simulink model "acrobot_sim_v3"  (R2013a)
settings: Solver=ode1  StartTime=0.0  StopTime=10.0  FixedStep=0.1  RelTol=1e-3
PreLoadFcn:
  | m1 = 1;
  | m2 = 1;
  | l1 = 1;
  | l2 = 1;
  | lc1 = l1/2;
  | lc2 = l2/2;
  | Ic1 = (lc1*lc1)/3;
  | Ic2 = (lc2*lc2)/3;
  | I1 = Ic1+m1*lc1*lc1;
  | I2 = Ic2+m2*lc2*lc2;
  | b1 = 0.4;
  | b2 = 0.4;
  | g = 9.8;
StartFcn:
  | m1 = 1;
  | m2 = 1;
  | l1 = 1;
  | l2 = 1;
  | lc1 = l1/2;
  | lc2 = l2/2;
  | Ic1 = (lc1*lc1)/3;
  | Ic2 = (lc2*lc2)/3;
  | I1 = Ic1+m1*lc1*lc1;
  | I2 = Ic2+m2*lc2*lc2;
  | b1 = 0.4;
  | b2 = 0.4;
  | g = 9.8;
libraries: mblibv1 x8, simulink x2
settings Model: Creator=nightling  LastModifiedBy=nightling
settings SimMechanicsCC: VisDuringSimulation=on

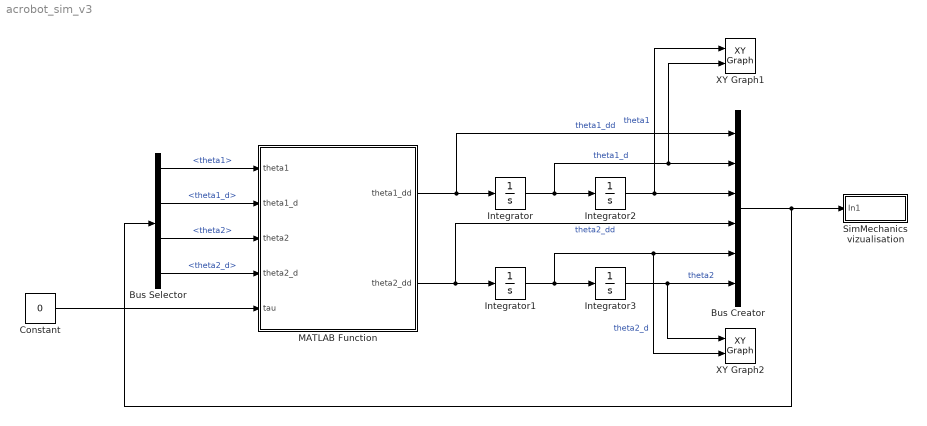
== system acrobot_sim_v3 ==
  Bus Creator : BusCreator  Inputs=6
  Bus Selector : BusSelector  OutputSignals=theta1,theta1_d,theta2,theta2_d
  Constant : Constant  Value=0
  Integrator : Integrator  InitialCondition=[0 ]
  Integrator1 : Integrator  InitialCondition=[0 ]
  Integrator2 : Integrator  InitialCondition=pi/2
  Integrator3 : Integrator  InitialCondition=[0 ]
  MATLAB Function : MATLAB Function  TreatAsAtomicUnit=on
  SimMechanics vizualisation : Subsystem
  XY Graph1 : simulink/Sinks/XY Graph  xmin=-1  xmax=1  ymin=-5  ymax=5  st=-1
  XY Graph2 : simulink/Sinks/XY Graph  xmin=-1  xmax=1  ymin=-5  ymax=5  st=-1
  wires:
  MATLAB Function/1(theta1_dd) -> Bus Creator/1, Integrator/1  "theta1_dd"
  MATLAB Function/2(theta2_dd) -> Integrator1/1, Bus Creator/4  "theta2_dd"
  Integrator/1 -> XY Graph1/2, Bus Creator/2, Integrator2/1  "theta1_d"
  Integrator1/1 -> Integrator3/1, XY Graph2/2, Bus Creator/5  "theta2_d"
  Integrator2/1 -> Bus Creator/3, XY Graph1/1  "theta1"
  Integrator3/1 -> XY Graph2/1, Bus Creator/6  "theta2"
  Constant/1 -> MATLAB Function/5(tau)
  Bus Creator/1 -> Bus Selector/1, SimMechanics vizualisation/1(In1)
  Bus Selector/1 -> MATLAB Function/1(theta1)  "<theta1>"
  Bus Selector/3 -> MATLAB Function/3(theta2)  "<theta2>"
  Bus Selector/2 -> MATLAB Function/2(theta1_d)  "<theta1_d>"
  Bus Selector/4 -> MATLAB Function/4(theta2_d)  "<theta2_d>"

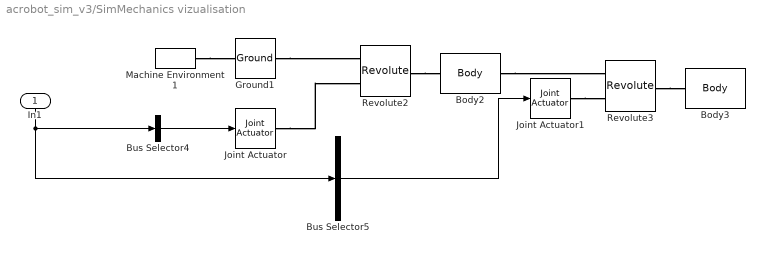
== system acrobot_sim_v3/SimMechanics vizualisation ==
  In1 : Inport
  Body2 : mblibv1/Bodies/Body  LConnTagsString=CS1  RConnTagsString=CS2  UpdateFromCAD=off  DialogClass=MechanicalBodyBlock  Mass=m1  MassUnits=kg  InertiaUnits=kg*m^2  Inertia=zeros(3)  Shape=Cylinder  ShapeDims=[1 1]  ShapeUnits=m  ShapeUse=false  Density=1  DensityUnits=kg/m^3  DensityUse=false  GraphicsMode=MACHINE_DEFAULT  BodyColorSelMode=COLORPALETTE  BodyColor=[0.043137 0.51765 0.78039]  AttachedToCS=CG  CG=Left$CG$[0 -l1/2 0]$CS1$CS1$m$[0 0 0]$Euler X-Y-Z$deg$WORLD$false$none  WorkingFrames=Left$CS1$[0 0 0]$Adjoining$Adjoining$m$[0 0 0]$Euler X-Y-Z$deg$WORLD$true$none#Right$CS2$[0 -l1 0]$CS1$CS1$m$[0 0 0]$Euler X-Y-Z$deg$WORLD$true$none  CGPos=[0 -l1/2 0]  CGRot=[0 0 0]  CS0Pos=[]  CS0Rot=[]  CS1Pos=[0 0 0]  CS1Rot=[0 0 0]  CS2Pos=[0 -l1 0]  CS2Rot=[0 0 0]  CS3Pos=[]  CS3Rot=[]  CS4Pos=[]  CS4Rot=[]  CS5Pos=[]  CS5Rot=[]  CS6Pos=[]  CS6Rot=[]  CS7Pos=[]  CS7Rot=[]  CS8Pos=[]  CS8Rot=[]  CS9Pos=[]  CS9Rot=[]  CS10Pos=[]  CS10Rot=[]  CS11Pos=[]  CS11Rot=[]  CS12Pos=[]  CS12Rot=[]  CS13Pos=[]  CS13Rot=[]  CS14Pos=[]  CS14Rot=[]  CS15Pos=[]  CS15Rot=[]  CS16Pos=[]  CS16Rot=[]  CS17Pos=[]  CS17Rot=[]  CS18Pos=[]  CS18Rot=[]  CS19Pos=[]  CS19Rot=[]  CS20Pos=[]  CS20Rot=[]
  Body3 : mblibv1/Bodies/Body  LConnTagsString=CS1  UpdateFromCAD=off  DialogClass=MechanicalBodyBlock  Mass=m2  MassUnits=kg  InertiaUnits=kg*m^2  Inertia=zeros(3)  Shape=Cylinder  ShapeDims=[1 1]  ShapeUnits=m  ShapeUse=false  Density=1  DensityUnits=kg/m^3  DensityUse=false  GraphicsMode=MACHINE_DEFAULT  BodyColorSelMode=COLORPALETTE  BodyColor=[0.043137 0.51765 0.78039]  AttachedToCS=CG  CG=Left$CG$[0 -l2/2 0]$CS1$CS1$m$[0 0 0]$Euler X-Y-Z$deg$WORLD$false$none  WorkingFrames=Left$CS1$[0 0 0]$Adjoining$Adjoining$m$[0 0 0]$Euler X-Y-Z$deg$WORLD$true$none#Right$CS2$[0 -l2 0]$CS1$CS1$m$[0 0 0]$Euler X-Y-Z$deg$WORLD$false$none  CGPos=[0 -l2/2 0]  CGRot=[0 0 0]  CS0Pos=[]  CS0Rot=[]  CS1Pos=[0 0 0]  CS1Rot=[0 0 0]  CS2Pos=[0 -l2 0]  CS2Rot=[0 0 0]  CS3Pos=[]  CS3Rot=[]  CS4Pos=[]  CS4Rot=[]  CS5Pos=[]  CS5Rot=[]  CS6Pos=[]  CS6Rot=[]  CS7Pos=[]  CS7Rot=[]  CS8Pos=[]  CS8Rot=[]  CS9Pos=[]  CS9Rot=[]  CS10Pos=[]  CS10Rot=[]  CS11Pos=[]  CS11Rot=[]  CS12Pos=[]  CS12Rot=[]  CS13Pos=[]  CS13Rot=[]  CS14Pos=[]  CS14Rot=[]  CS15Pos=[]  CS15Rot=[]  CS16Pos=[]  CS16Rot=[]  CS17Pos=[]  CS17Rot=[]  CS18Pos=[]  CS18Rot=[]  CS19Pos=[]  CS19Rot=[]  CS20Pos=[]  CS20Rot=[]
  Bus Selector4 : BusSelector  OutputSignals=theta1,theta1_d,theta1_dd  OutputAsBus=on
  Bus Selector5 : BusSelector  OutputSignals=theta2,theta2_d,theta2_dd  OutputAsBus=on
  Ground1 : mblibv1/Bodies/Ground  UpdateFromCAD=off  LeftPortType=env  RightPortType=workingframe  PhysicalDomain=Mechanical  DialogClass=GroundBlock  CoordPosition=[1 0 0]  CoordPositionUnits=m  StateVectorMgrId=6  MachineId=[7 0]  ShowEnvPort=on
  Joint Actuator : mblibv1/Sensors &  Actuators/Joint Actuator  UpdateFromCAD=off  PhysicalDomain=Mechanical  PortType=blob  ActuationStyle=Motion  AngleUnits=rad  ArcVelocityUnits=rad/s  ArcAccelerationUnits=rad/s^2  CoordPositionUnits=m  VelocityUnits=m/s  AccelerationUnits=m/s^2  ForceUnits=N  TorqueUnits=N*m  ActiveIO=on  Width=3  DialogClass=MechanicalActuatorBlock  Primitive=R1  ReferenceFrame=Absolute (World)
  Joint Actuator1 : mblibv1/Sensors &  Actuators/Joint Actuator  UpdateFromCAD=off  PhysicalDomain=Mechanical  PortType=blob  ActuationStyle=Motion  AngleUnits=rad  ArcVelocityUnits=rad/s  ArcAccelerationUnits=rad/s^2  CoordPositionUnits=m  VelocityUnits=m/s  AccelerationUnits=m/s^2  ForceUnits=N  TorqueUnits=N*m  ActiveIO=on  Width=3  DialogClass=MechanicalActuatorBlock  Primitive=R1  ReferenceFrame=Absolute (World)
  Machine Environment1 : mblibv1/Bodies/Machine Environment  PortType=env  PhysicalDomain=Mechanical  DialogTemplateClass=MECH.MachineEnvironment  SyncWhenCopied=off  Gravity=[0 -9.81 0]  GravityUnits=m/s^2  GravityAsSignal=off  Dimensionality=Auto-detect  AnalysisType=Forward dynamics  LinearAssemblyTolerance=1e-3  LinearAssemblyToleranceUnits=m  AngularAssemblyTolerance=1e-3  AngularAssemblyToleranceUnits=rad  ConstraintSolverType=Stabilizing  ConstraintRelTolerance=1e-4  ConstraintAbsTolerance=1e-4  UseRobustSingularityHandling=off  RedundancyAnalysisToleranceType=Automatically select tolerance  RedundancyAnalysisTolerance=1e-14  StatePerturbationType=Fixed  PerturbationSize=1e-5  VisualizeMachine=on  BodyVisualizationType=Use model default body geometries  BodyColorSelMode=Use model default  DefaultBodyColor=[1 0 0]
  Revolute2 : mblibv1/Joints/Revolute  LConnTagsString=__newl0|SA1  RConnTagsString=__newr0  UpdateFromCAD=off  NumSAPorts=1  CutJoint=off  MarkAsCut=off  Primitives=prismatic  PrimitiveProps=R1$World$[0 0 1]$revolute  DialogClass=JointBlock  R1Axis=[0 0 1]
  Revolute3 : mblibv1/Joints/Revolute  LConnTagsString=__newl0|SA1  RConnTagsString=__newr0  UpdateFromCAD=off  NumSAPorts=1  CutJoint=off  MarkAsCut=off  Primitives=prismatic  PrimitiveProps=R1$World$[0 0 1]$revolute  DialogClass=JointBlock  R1Axis=[0 0 1]
  wires:
  Bus Selector4/1 -> Joint Actuator/1
  In1/1 -> Bus Selector5/1, Bus Selector4/1
  Bus Selector5/1 -> Joint Actuator1/1
  connections:
  Revolute2/RConn1 -- Body2/LConn1
  Body2/RConn1 -- Revolute3/LConn1
  Revolute3/RConn1 -- Body3/LConn1
  Machine Environment1/RConn1 -- Ground1/LConn1
  Ground1/RConn1 -- Revolute2/LConn1
  Joint Actuator/RConn1 -- Revolute2/LConn2
  Joint Actuator1/RConn1 -- Revolute3/LConn2

== matlab function acrobot_sim_v3/MATLAB Function ==
  data: theta1 input; theta1_dd output; theta1_d input; theta2 input; theta2_d input; theta2_dd output; tau input
function [theta1_dd, theta2_dd] = Acrobot(theta1, theta1_d, theta2, theta2_d, tau)
%#codegen
    
    coder.extrinsic('AcrobotDynamics');
    theta1_dd = 0;
    theta2_dd = 0;
    
    [theta1_dd,theta2_dd] = AcrobotDynamics(theta1, theta1_d, theta2, theta2_d, tau);
